simulink model "Simpel_Model_2"  (R2016a)
settings: Solver=VariableStepAuto  StartTime=0.0  StopTime=50.0  RelTol=1e-3
values from neighbouring files (symbols this model uses):
  K = 651/12    (= 54.25)    [Model.m]    (also in PID_test.m = 96.2958333333; Rlocus.m = 0.0274)
  T = 0.014    [Model.m]    (also in PID_test.m = 0.12)
settings Model: Creator=Kristian  LastModifiedBy=Kristian

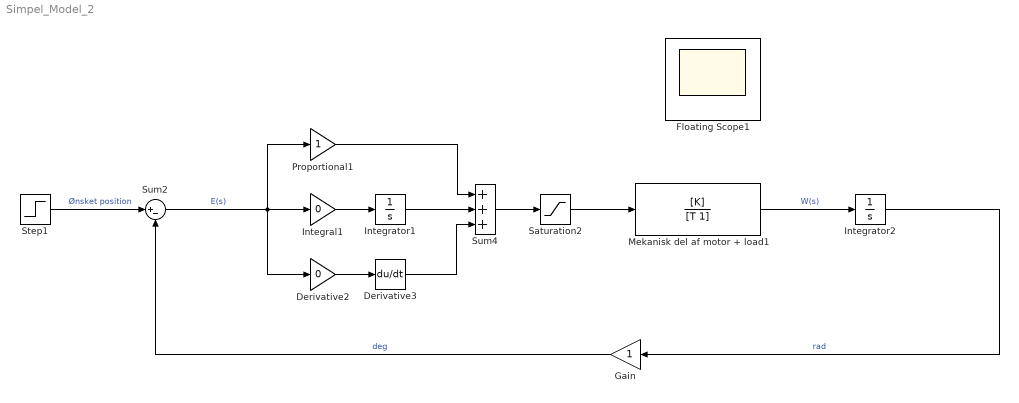
== system Simpel_Model_2 ==
  Derivative2 : Gain  Gain=0  OutMin=-5  OutMax=5
  Derivative3 : Derivative
  Floating Scope1 : Scope
      settings: Floating=on
  Gain : Gain
  Integral1 : Gain  Gain=0  OutMin=-5  OutMax=5
  Integrator1 : Integrator
  Integrator2 : Integrator
  Mekanisk del af motor + load1 : TransferFcn  Numerator=[K]  Denominator=[T 1]
  Proportional1 : Gain  OutMin=-5  OutMax=5
  Saturation2 : Saturate  UpperLimit=12  LowerLimit=-12
  Step1 : Step  After=10  SampleTime=0
  Sum2 : Sum  Inputs=|+-
  Sum4 : Sum  Inputs=+++
  wires:
  Mekanisk del af motor + load1/1 -> Integrator2/1  "W(s)"
  Gain/1 -> Sum2/2  "deg"
  Step1/1 -> Sum2/1  "Ønsket position"
  Integrator2/1 -> Gain/1  "rad"
  Sum2/1 -> Integral1/1, Derivative2/1, Proportional1/1  "E(s)"
  Proportional1/1 -> Sum4/1
  Sum4/1 -> Saturation2/1
  Integral1/1 -> Integrator1/1
  Integrator1/1 -> Sum4/2
  Derivative2/1 -> Derivative3/1
  Derivative3/1 -> Sum4/3
  Saturation2/1 -> Mekanisk del af motor + load1/1
